simulink model "Drivetrain_2Track"  (R2020a)
settings: Solver=VariableStepAuto  StartTime=0.0  StopTime=10.0  MaxStep=0.2  RelTol=1e-3
values from neighbouring files (symbols this model uses):
  Engine_inertia = 0.0896    [Properties.sldd]
  Transmission_ratios : value not decoded    [Properties.sldd]
undefined symbols (not defined in the file or in its folder): Initial_omega
libraries: autolibshareddiff x1
settings Model: DataDictionary=Properties.sldd  Creator=yafta  LastModifiedBy=Matthew
settings ModelReferenceCC: ModelReferenceMinAlgLoopOccurrences=on

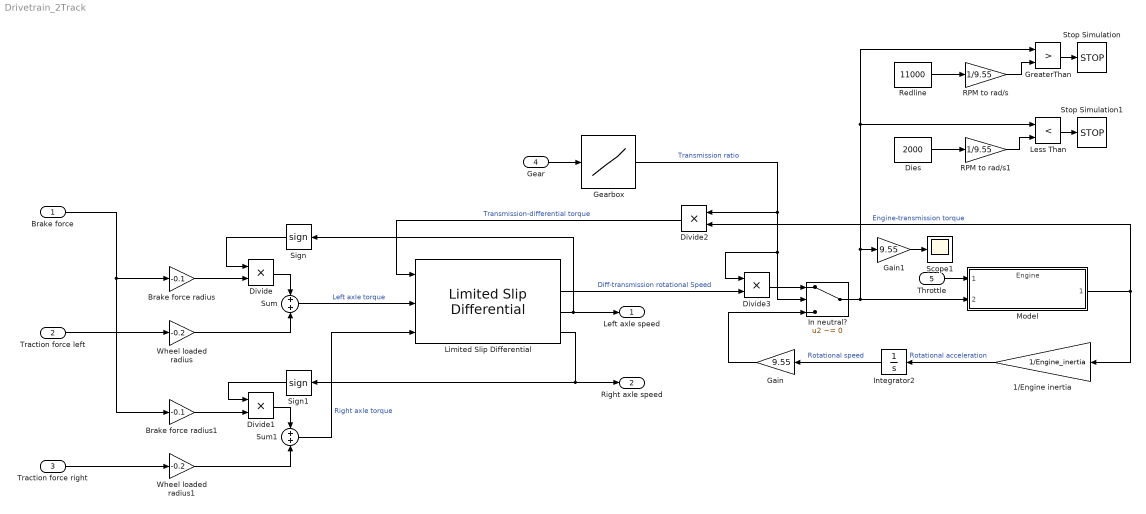
== system Drivetrain_2Track ==
  Brake force : Inport
  Traction force left : Inport  Port=2
  Traction force right : Inport  Port=3
  Gear : Inport  Port=4
  Throttle : Inport  Port=5
  1/Engine inertia : Gain  Gain=1/Engine_inertia
  Brake force radius : Gain  Gain=-0.1
  Brake force radius1 : Gain  Gain=-0.1
  Dies : Constant  Value=2000
  Divide{,1..3} (4 alike) : Product  Inputs=**
  Gain : Gain  Gain=9.55
  Gain1 : Gain  Gain=9.55
  Gearbox : Lookup_n-D  NumberOfTableDimensions=1  BreakpointsForDimension1=Transmission_ratios(:,1)  BreakpointsForDimension1DataTypeStr=int8  BeginIndexSearchUsingPreviousIndexResult=on  Table=Transmission_ratios(:,2)  TableMin=0  TableMax=5  TableDataTypeStr=double  InterpMethod=Flat  DiagnosticForOutOfRangeInput=Error  InternalRulePriority=Speed  OutDataTypeStr=double  RndMeth=Simplest  InputSameDT=on
  GreaterThan : RelationalOperator  Operator=>  OutDataTypeStr=boolean  RndMeth=Simplest
  In neutral? : Switch  Criteria=u2 ~= 0
  Integrator2 : Integrator  InitialCondition=4000/9.55
  Less Than : RelationalOperator  Operator=<  OutDataTypeStr=boolean  RndMeth=Simplest
  Limited Slip Differential : autolibshareddiff/Limited Slip Differential  DiffEffModelPopup=Constant  InterpMethod=Linear point-slope  extTamb=off  shaftSwitchMask=To the left of center-line  Ndiff=40/11  Jd=Engine_inertia  bd=1e-3  Jw1=Wheel_inertia  bw1=0  Jw2=Wheel_inertia  bw2=0  omegaw1o=-Initial_omega  omegaw2o=-Initial_omega  eta=1  eta_tbl=reshape([0.64 0.76 0.8 0.81 0.83 0.84 0.84 0.56 0.73 0.78 0.8 0.83 0.84 0.84 0.54 0.71 0.77 0.8 0.82 0.84 0.84 0.53 0.71 0.77 0.8 0.83 0.84 0.84 0.51 0.71 0.77 0.8 0.83 0.84 0.85 0.52 0.7 0.77 0.8 0.83 0.84 0.85 0.51 0.71 0.76 0.79 0.83 0.84 0.85 0.5 0.69 0.76 0.79 0.82 0.84 0.85 0.45 0.68 0.75 0.78 0.82 0.84 0.85 0.43 0.67 0.74 0.78 0.81 0.83 0.84 0.38 0.63 0.71 0.75 0.8 0.82 0.83 0.81 0.86 0.88 0.89 0.89 0.89 0.9 0.77 0.85 0.87 0.88 0.89 0.9 0.9 0.72 0.82 0.86 0.87 0.88 0.89 0.9 0.68 0.8 0.84 0.86 0.88 0.89 0.89 0.67 0.8 0.84 0.86 0.88 0.89 0.9 0.67 0.8 0.84 0.86 0.88 0.89 0.9 0.65 0.8 0.84 0.86 0.88 0.89 0.9 0.64 0.79 0.83 0.86 0.88 0.89 0.9 0.63 0.78 0.83 0.86 0.88 0.89 0.9 0.59 0.76 0.82 0.85 0.87 0.89 0.9 0.53 0.73 0.8 0.83 0.86 0.88 0.89], 7, 11, 2)  Trq_bpts=[25, 50, 75, 100, 150, 200, 250]  omega_bpts=[52.4 78.5 105 131 157 183 209 262 314 419 524]  Temp_bpts=[290 358]  Tamb=297.15  couplingType=Pre-loaded ideal clutch  Ndisks=4  Reff=.20  Fc=500  muc=[.16 0.13 0.115 0.11 0.105 0.1025 0.10125]  dw=[0 10 20 40 60 80 100]  Tdw=[-100, -90, -50, -5, 0, 5, 50, 90, 100]  dwT=[-200, -175, -100, - 50, 0, 50, 100, 175, 200]  TTin=[-200 -175 -100 - 50 0 50 100 175 200]  Tin=[-200 -175 -100 - 50 0 50 100 175 200]  tauC=.01  IdealInterpMethod=Linear point-slope  IdealExtrapMethod=Clip  TdwInterpMethod=Linear point-slope  TdwExtrapMethod=Clip  TTinInterpMethod=Linear point-slope  TTinExtrapMethod=Clip  maxAbsSpd=5e3  aMode=2
      settings: SourceProductBaseCode=PW,MT,VE,VP
  Model : ModelReference  ModelNameDialog=Engine  SimulationMode=Normal  ModelReferenceVersion=1.8
  RPM to rad/s : Gain  Gain=1/9.55
  RPM to rad/s1 : Gain  Gain=1/9.55
  Redline : Constant  Value=11000
  Scope1 : Scope
  Sign : Signum
  Sign1 : Signum
  Stop Simulation : Stop
  Stop Simulation1 : Stop
  Sum : Sum  Inputs=2
  Sum1 : Sum  Inputs=2
  Wheel loaded radius : Gain  Gain=-0.2
  Wheel loaded radius1 : Gain  Gain=-0.2
  Left axle speed : Outport
  Right axle speed : Outport  Port=2
  wires:
  Gearbox/1 -> Divide2/1, Divide3/1, In neutral?/2  "Transmission ratio"
  Model/1 -> 1/Engine inertia/1, Divide2/2  "Engine-transmission torque"
  Limited Slip Differential/2 -> Divide3/2  "Diff-transmission rotational Speed"
  Integrator2/1 -> Gain/1  "Rotational speed"
  Traction force left/1 -> Wheel loaded radius/1
  Gear/1 -> Gearbox/1
  Divide2/1 -> Limited Slip Differential/1  "Transmission-differential torque"
  1/Engine inertia/1 -> Integrator2/1  "Rotational acceleration"
  Traction force right/1 -> Wheel loaded radius1/1
  Brake force/1 -> Brake force radius1/1, Brake force radius/1
  Wheel loaded radius/1 -> Sum/2
  Sum/1 -> Limited Slip Differential/2  "Left axle torque"
  Brake force radius1/1 -> Divide1/2
  Wheel loaded radius1/1 -> Sum1/2
  Sum1/1 -> Limited Slip Differential/3  "Right axle torque"
  Sign/1 -> Divide/1
  Brake force radius/1 -> Divide/2
  Divide/1 -> Sum/1
  Divide1/1 -> Sum1/1
  Limited Slip Differential/3 -> Sign/1, Left axle speed/1
  Limited Slip Differential/4 -> Sign1/1, Right axle speed/1
  Sign1/1 -> Divide1/1
  Divide3/1 -> In neutral?/1
  Throttle/1 -> Model/1
  Redline/1 -> RPM to rad/s/1
  GreaterThan/1 -> Stop Simulation/1
  RPM to rad/s/1 -> GreaterThan/2
  Less Than/1 -> Stop Simulation1/1
  Dies/1 -> RPM to rad/s1/1
  RPM to rad/s1/1 -> Less Than/2
  Gain1/1 -> Scope1/1
  In neutral?/1 -> Model/2, GreaterThan/1, Less Than/1, Gain1/1
  Gain/1 -> In neutral?/3
